simulink model "Dynamics"  (R2017a)
settings: Solver=VariableStepAuto  StartTime=0.0  StopTime=100  RelTol=1e-3
(part 1 of 8)
settings Model: Creator=Aaa  LastModifiedBy=Aaa

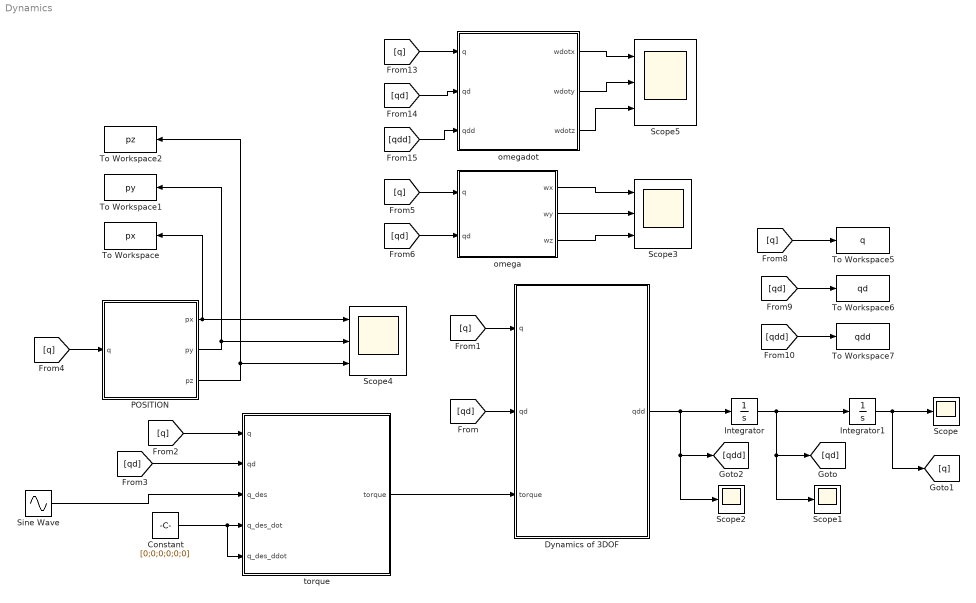
== system Dynamics ==
  Constant : Constant  Value=[0;0;0;0;0;0]
  Dynamics of 3DOF : MATLAB Function  TreatAsAtomicUnit=on
  Integrator : Integrator  InitialCondition=[0;0;0;0;0;0]
  Integrator1 : Integrator  InitialCondition=[1;1;1;1;1;1]
  POSITION : MATLAB Function  TreatAsAtomicUnit=on
  Scope : Scope
  Scope1 : Scope
  Scope2 : Scope
  Scope3 : Scope  NumInputPorts=3
  Scope4 : Scope  NumInputPorts=3
  Scope5 : Scope  NumInputPorts=3
  Sine Wave : Sin  SampleTime=0
  To Workspace : ToWorkspace  VariableName=px  SampleTime=-1
  To Workspace1 : ToWorkspace  VariableName=py  SampleTime=-1
  To Workspace2 : ToWorkspace  VariableName=pz  SampleTime=-1
  To Workspace5 : ToWorkspace  VariableName=q  SampleTime=-1
  To Workspace6 : ToWorkspace  VariableName=qd  SampleTime=-1
  To Workspace7 : ToWorkspace  VariableName=qdd  SampleTime=-1
  omega : MATLAB Function  TreatAsAtomicUnit=on
  omegadot : MATLAB Function  TreatAsAtomicUnit=on
  torque : MATLAB Function  TreatAsAtomicUnit=on
  wires:
  [qdd] -> omegadot/3(qdd)
  omegadot/2(wdoty) -> Scope5/2
  omega/2(wy) -> Scope3/2
  omegadot/3(wdotz) -> Scope5/3
  [q] -> omegadot/1(q)
  omega/1(wx) -> Scope3/1
  POSITION/3(pz) -> To Workspace2/1, Scope4/3
  omegadot/1(wdotx) -> Scope5/1
  Sine Wave/1 -> torque/3(q_des)
  [qd] -> To Workspace6/1
  [qd] -> omegadot/2(qd)
  [qd] -> Dynamics of 3DOF/2(qd)
  Constant/1 -> torque/5(q_des_ddot), torque/4(q_des_dot)
  [q] -> Dynamics of 3DOF/1(q)
  [q] -> torque/1(q)
  [q] -> To Workspace5/1
  POSITION/1(px) -> To Workspace/1, Scope4/1
  [q] -> POSITION/1(q)
  Integrator/1 -> Integrator1/1, Scope1/1, [qd]
  [qd] -> torque/2(qd)
  [qd] -> omega/2(qd)
  omega/3(wz) -> Scope3/3
  [qdd] -> To Workspace7/1
  Dynamics of 3DOF/1(qdd) -> [qdd], Scope2/1, Integrator/1
  torque/1(torque) -> Dynamics of 3DOF/3(torque)
  POSITION/2(py) -> To Workspace1/1, Scope4/2
  Integrator1/1 -> [q], Scope/1
  [q] -> omega/1(q)
